simulink model "untitled"  (R2021a)
settings: Solver=FixedStepDiscrete  StartTime=0.0  StopTime=inf  FixedStep=0.1  RelTol=1e-3  EnableMultiTasking=on
settings Model: SILPILModeSetting=veronly  EnablePacing=on  ExtModeTrigDuration=2  Creator=smrh1  LastModifiedBy=Abbas
settings SolverCC: AlgebraicLoopSolver=TrustRegion  AutoInsertRateTranBlk=on
settings OptimizationCC: LifeSpan=inf
settings DebuggingCC: SFUnexpectedBacktrackingDiag=warning  SFNoUnconditionalDefaultTransitionDiag=warning  SFExecutionAtInitializationDiag=none  ArithmeticOperatorsInVariantConditions=warning
settings SFSimCC: SimUseLocalCustomCode=off  CustomCodeUndefinedFunction=UseInterfaceOnly
settings RTWCC: RTWUseLocalCustomCode=off  BuildConfiguration=Faster Runs
settings CodeAppCC: StateflowObjectComments=on
settings GRTTargetCC: TargetLangStandard=C89/C90 (ANSI)
settings ConfigComp: CovMetricSettings=dw  CovSaveCumulativeToWorkspaceVar=on  CovSaveSingleToWorkspaceVar=on  CovExternalEMLEnable=off

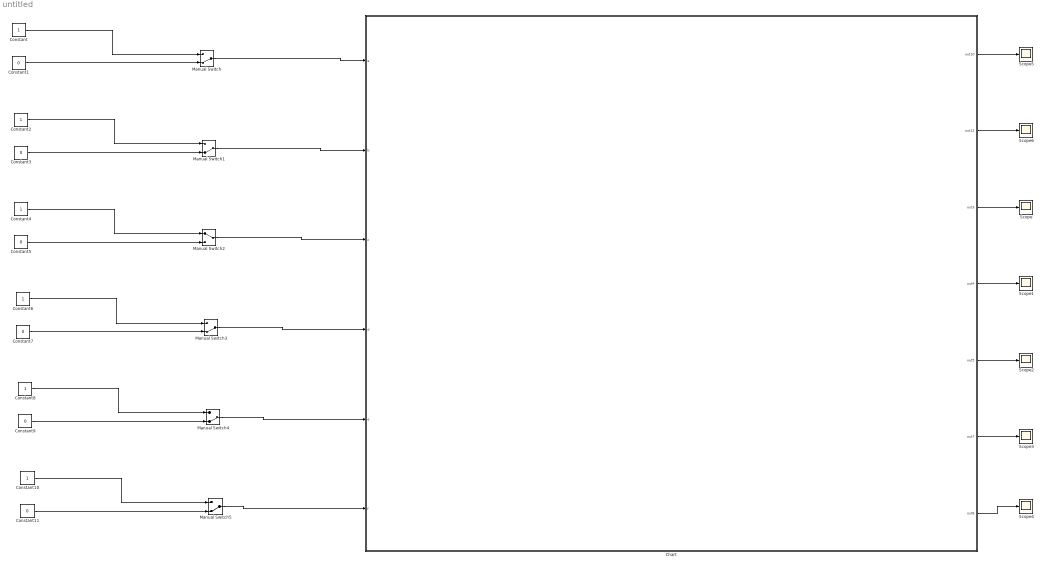
== system untitled ==
  Chart : Stateflow chart  TreatAsAtomicUnit=on
  Constant{,2,4,6,8,10} (6 alike) : Constant
  Constant{1,3,5,7,9,11} (6 alike) : Constant  Value=0
  Manual Switch{,1,3..5} (5 alike) : ManualSwitch  CurrentSetting=0
  Manual Switch2 : ManualSwitch
  Scope{,1..6} (7 alike) : Scope
  wires:
  Constant/1 -> Manual Switch/1
  Constant1/1 -> Manual Switch/2
  Manual Switch/1 -> Chart/1(a)
  Constant2/1 -> Manual Switch1/1
  Constant3/1 -> Manual Switch1/2
  Manual Switch1/1 -> Chart/2(b)
  Constant4/1 -> Manual Switch2/1
  Constant5/1 -> Manual Switch2/2
  Manual Switch2/1 -> Chart/3(c)
  Manual Switch3/1 -> Chart/4(d)
  Constant7/1 -> Manual Switch3/2
  Constant6/1 -> Manual Switch3/1
  Manual Switch4/1 -> Chart/5(e)
  Constant8/1 -> Manual Switch4/1
  Constant9/1 -> Manual Switch4/2
  Constant10/1 -> Manual Switch5/1
  Constant11/1 -> Manual Switch5/2
  Manual Switch5/1 -> Chart/6(f)
  Chart/3(out3) -> Scope/1
  Chart/4(out4) -> Scope1/1
  Chart/5(out5) -> Scope2/1
  Chart/6(out7) -> Scope3/1
  Chart/7(out8) -> Scope4/1
  Chart/1(out10) -> Scope5/1
  Chart/2(out12) -> Scope6/1

== stateflow chart untitled/Chart ==
  state state2
    state state6
      state d [parallel]
        settings: executionOrder=3
        state state8
        state state9
        state9 -> state8 : [a==1 & hasChanged(a)]{out8 =1}
        state8 -> state9 : [b==1& hasChanged(b)]{out8 =0}
        (default) -> state9
      state e [parallel]
        settings: executionOrder=1
        state state10
        state state11
        state11 -> state10 : [c==1& hasChanged(c)]{out10 =1}
        state10 -> state11 : [c==1& hasChanged(c)]{out10 =0}
        (default) -> state11
      state f [parallel]
        settings: executionOrder=2
        state state12
        state state13
        state13 -> state12 : [c==1& hasChanged(c)]{out12 =1}
        state12 -> state13 : [a==1& hasChanged(a)]{out12 =0}
        (default) -> state13
    state state7
    state7 -> state6 [order 2] : [e==1& hasChanged(e)]{out7 =0}
    state6 -> state7 : [d==1& hasChanged(d)]{out7 =1}
    (default) -> state6
  state state1
    (history)
    state state4
    state state5
    (default) -> state4 : {out4 =1}
    state5 -> state4 : [a==1& hasChanged(a)]{out4 =1;out5 =0}
    state4 -> state5 : [b==1& hasChanged(b)]{out4 =0;out5 =1}
  state state3
  (default) -> state1
  state1 -> state2 [order 1] : [f==1]
  state3 -> state5 : [e==1& hasChanged(e)]{out3 =0}
  state7 -> state1 [order 1] : [b==1& hasChanged(b)]{out7 =0}
  state1 -> state3 [order 2] : [d==1& hasChanged(d)]{out3 =1}
  data: a input; b input; c input; d input; e input; f input; out10 output double; out12 output double; out3 output double; out4 output double; out5 output double; out7 output double; out8 output double
